simulink library "vmc"  (R2021b)
settings: Solver=VariableStepAuto  StartTime=0.0  StopTime=10.0  RelTol=1e-3
undefined symbols (not defined in the file or in its folder): AVMC_ACCDeltaTqIGain4OVRD_X_kph, AVMC_ACCDeltaTqIGain4OVRD_Y_mps2, AVMC_ACCDeltaTqIGain_X_kph, AVMC_ACCDeltaTqIGain_Y_mps2, AVMC_ACCDeltaTqPGain_X_kph, AVMC_ACCDeltaTqPGain_Y_kph, AVMC_ACCLongSteadyCtrl_X_kph, AVMC_ADSPosGFBDeltaTq_X_kph, AVMC_ADSPosGFBDeltaTq_Y_mps2, AVMC_AggressJerkPCT4AT_X_kph, AVMC_AggressJerkPCT_X_kph, AVMC_AggressLimitPCT4AT_X_kph, AVMC_AggressLimitPCT_X_kph, AVMC_CCLongSteadyCtrl_X_kph, AVMC_DISCDeltaTqIGain_X_kph, AVMC_DISCDeltaTqIGain_Y_mps2, AVMC_DISCDeltaTqPGain_X_kph, AVMC_DISCDeltaTqPGain_Y_kph, AVMC_ESCRegenOut_X_kph, AVMC_ESCRegenOut_Y_Deg, AVMC_ESCRegenOutEnSpd_X_Deg, AVMC_ISOAccLimit_X_mps, AVMC_ISODecLimit_X_mps, AVMC_ISOJerk_X_mps, AVMC_LatESCRegenOut_X_kph, AVMC_LatESCRegenOut_Y_Deg, AVMC_LongAccDeadZone_X_kph, AVMC_LongAccFiltTsforP2_X_Gps, AVMC_MCPresBaseTq_X_bar, AVMC_MSALongSteadyCtrl_X_kph, AVMC_MSAPedalOvrd_X_kph, AVMC_MSASpdBand_X_kph, AVMC_MSATqDownEndTq_X_kph, AVMC_MSATqDownTime_X_kph, AVMC_OPDDisSlideRate_X_Deg, AVMC_OVRD2ActSR2FCMCMD_X_mps2, AVMC_PedalTqRWhlRatio_X_Nm, AVMC_PedalTqRWhlRatio_Y_gps, AVMC_PedalTqRWhlSlipGain_X_rat, AVMC_PedalTqRWhlSlipGain_Y_kph, AVMC_PedalTqRWhSTRGGain_X_deg, AVMC_PedalTqRWhSTRGGain_Y_kph, AVMC_RDCDetectTime_X_kph, AVMC_RDCDetectTime_Y_pct, AVMC_RDCEnSlideRate_X_Deg, AVMC_RearWhlTqRatio_X_Nm, AVMC_RearWhlTqRatio_Y_gps, AVMC_RearWhlTqSlipGain_X_rat, AVMC_RearWhlTqSlipGain_Y_kph, AVMC_RearWhlTqSTRGGain_X_deg, AVMC_RearWhlTqSTRGGain_Y_kph, AVMC_ReqBrkJoinDecSR_X_mps2, AVMC_SoftJerkPCT_X_kph, AVMC_SoftLimitPCT_X_kph, AVMC_StESCYaw_X_kph, AVMC_StESCYaw_Y_Deg, AVMC_StESCYawCom_X_kph, AVMC_StESCYawCom_Y_Gps, AVMC_TMSpdBaseTq_X_rpm, AVMC_VehHoldDecCtrlTime2_X_kph ... (+411)
libraries: hcu_lib x108, simulink x82, tqr x1, simulink_extras x1
(part 12 of 14)

== system vmc/VMC/VMC/SpeedArbitration/Response Gain ==
  VDSC_DISCTurn_flg : Inport
  VVMC_FeatArbitrSta_enum : Inport  Port=2
  VVMC_FeatReqSpd_kph : Inport  Port=3
  VVMC_MeterIndSpeedForCalcu_kph : Inport  Port=4
  VINP_VehSpeed_kph : Inport  Port=5
  VDSC_AutoTurnMode_flg : Inport  Port=6
  VDSC_DISCTargetSpd_kph : Inport  Port=7
  Abs : Abs
  Add : Sum  Inputs=-+
  Add4 : Sum
  Constant1 : Constant  Value=KVMC_Veh2MeterSpdFactor_enum
  Constant13 : Constant  Value=ENUM_FEATARBITRSTA_DISC
  Constant{15,29,31,33,35} (5 alike) : Constant  Value=ZERO_FLOAT
  Constant16 : Constant  Value=ENUM_DISCTURN_ACTIVE
  Constant18 : Constant  Value=ENUM_FEATARBITRSTA_ACCDISC
  Constant2 : Constant  Value=ENUM_FEATARBITRSTA_CC
  Constant23 : Constant  Value=KVMC_Veh2MeterSpdOffset_enum
  Constant28 : Constant  Value=KVMC_Veh2MeterSpdLoFactor_enum
  Constant3 : Constant  Value=ENUM_FEATARBITRSTA_MSA
  Constant{30,32,34,36} (4 alike) : Constant  Value=HUNDRED
  Constant4 : Constant  Value=TRUE
  Constant5 : Constant  Value=KVMC_MSAResponseAGSV_flg
  Divide5 : Product  Inputs=**
  Divide8 : Product  Inputs=**
  MVMC_AggressJerkPCT4AT_pct : Lookup_n-D  NumberOfTableDimensions=1  BreakpointsForDimension1=AVMC_AggressJerkPCT4AT_X_kph  Table=MVMC_AggressJerkPCT4AT_Y_pct  InternalRulePriority=Speed  RndMeth=Simplest  InputSameDT=on
  MVMC_AggressJerkPCT_pct : Lookup_n-D  NumberOfTableDimensions=1  BreakpointsForDimension1=AVMC_AggressJerkPCT_X_kph  Table=MVMC_AggressJerkPCT_Y_pct  InternalRulePriority=Speed  RndMeth=Simplest  InputSameDT=on
  MVMC_AggressJerkPCT_pct1 : Lookup_n-D  NumberOfTableDimensions=1  BreakpointsForDimension1=AVMC_AggressJerkPCT_X_kph  Table=MVMC_AggressJerkPCT_Y_pct  InternalRulePriority=Speed  RndMeth=Simplest  InputSameDT=on
  MVMC_AggressLimitPCT4AT_pct : Lookup_n-D  NumberOfTableDimensions=1  BreakpointsForDimension1=AVMC_AggressLimitPCT4AT_X_kph  Table=MVMC_AggressLimitPCT4AT_Y_pct  InternalRulePriority=Speed  RndMeth=Simplest  InputSameDT=on
  MVMC_AggressLimitPCT_pct : Lookup_n-D  NumberOfTableDimensions=1  BreakpointsForDimension1=AVMC_AggressLimitPCT_X_kph  Table=MVMC_AggressLimitPCT_Y_pct  InternalRulePriority=Speed  RndMeth=Simplest  InputSameDT=on
  MVMC_AggressLimitPCT_pct1 : Lookup_n-D  NumberOfTableDimensions=1  BreakpointsForDimension1=AVMC_AggressLimitPCT_X_kph  Table=MVMC_AggressLimitPCT_Y_pct  InternalRulePriority=Speed  RndMeth=Simplest  InputSameDT=on
  MVMC_SoftJerkPCT_pct : Lookup_n-D  NumberOfTableDimensions=1  BreakpointsForDimension1=AVMC_SoftJerkPCT_X_kph  Table=MVMC_SoftJerkPCT_Y_pct  InternalRulePriority=Speed  RndMeth=Simplest  InputSameDT=on
  MVMC_SoftLimitPCT_pct : Lookup_n-D  NumberOfTableDimensions=1  BreakpointsForDimension1=AVMC_SoftLimitPCT_X_kph  Table=MVMC_SoftLimitPCT_Y_pct  InternalRulePriority=Speed  RndMeth=Simplest  InputSameDT=on
  Relational Operator : RelationalOperator  Operator=>  OutDataTypeStr=boolean  RndMeth=Simplest
  Relational Operator1 : RelationalOperator  Operator=>  OutDataTypeStr=boolean  RndMeth=Simplest
  Response Gain : Stateflow chart  TreatAsAtomicUnit=on
  Saturation Dynamic{1..4} (4 alike) : simulink/Discontinuities/Saturation Dynamic  OutMin=[]  OutMax=[]  OutDataTypeStr=Inherit: Same as second input  OutDataType=fixdt(1, 16)  OutScaling=2^-10  DoSatur=off
  Switch : Switch  Criteria=u2 > Threshold  Threshold=KVMC_Veh2MeterSpdLoBdy_kph
  Switch{1..4} (4 alike) : Switch  Criteria=u2 > Threshold
  VVMC_JerkPCT_pct : Outport
  VVMC_LimitPCT_pct : Outport  Port=2
  wires:
  Switch/1 -> Add/1
  VINP_VehSpeed_kph/1 -> [VINP_VehSpeed_kph]
  Abs/1 -> MVMC_SoftLimitPCT_pct/1, MVMC_AggressLimitPCT_pct/1, MVMC_AggressLimitPCT4AT_pct/1, MVMC_AggressLimitPCT_pct1/1
  Add/1 -> Abs/1
  [VVMC_FeatReqSpd_kph] -> Add/2
  VVMC_FeatReqSpd_kph/1 -> [VVMC_FeatReqSpd_kph]
  Switch1/1 -> Saturation Dynamic3/2
  Saturation Dynamic1/1 -> [VVMC_SoftLimitPCT_pct]  "VVMC_SoftLimitPCT_pct"
  Saturation Dynamic2/1 -> [VVMC_AggressJerkPCT_pct]  "VVMC_AggressJerkPCT_pct"
  Saturation Dynamic4/1 -> [VVMC_SoftJerkPCT_pct]  "VVMC_SoftJerkPCT_pct"
  [VVMC_MeterIndSpeedForCalcu_kph] -> MVMC_SoftJerkPCT_pct/1, MVMC_AggressJerkPCT4AT_pct/1, MVMC_AggressJerkPCT_pct/1, MVMC_AggressJerkPCT_pct1/1
  VVMC_MeterIndSpeedForCalcu_kph/1 -> [VVMC_MeterIndSpeedForCalcu_kph]
  Constant18/1 -> Response Gain/11(ENUM_FEATARBITRSTA_ACCDISC)
  Constant16/1 -> Response Gain/10(ENUM_DISCTURN_ACTIVE)
  Constant15/1 -> Response Gain/9(ZERO_FLOAT)
  Constant13/1 -> Response Gain/7(ENUM_FEATARBITRSTA_DISC)
  [VVMC_LimitPCT_pct] -> VVMC_LimitPCT_pct/1
  [VVMC_JerkPCT_pct] -> VVMC_JerkPCT_pct/1
  [VVMC_AggressLimitPCT_pct] -> Response Gain/6(VVMC_AggressLimitPCT_pct)
  [VVMC_SoftLimitPCT_pct] -> Response Gain/5(VVMC_SoftLimitPCT_pct)
  [VVMC_AggressJerkPCT_pct] -> Response Gain/4(VVMC_AggressJerkPCT_pct)
  [VVMC_SoftJerkPCT_pct] -> Response Gain/3(VVMC_SoftJerkPCT_pct)
  [VVMC_FeatArbitrSta_enum] -> Response Gain/2(VVMC_FeatArbitrSta_enum)
  VVMC_FeatArbitrSta_enum/1 -> [VVMC_FeatArbitrSta_enum]
  VDSC_DISCTurn_flg/1 -> [VDSC_DISCTurn_flg]
  Response Gain/2(VVMC_LimitPCT_pct) -> [VVMC_LimitPCT_pct]
  [VDSC_DISCTurn_flg] -> Response Gain/1(VDSC_DISCTurn_flg)
  Response Gain/1(VVMC_JerkPCT_pct) -> [VVMC_JerkPCT_pct]
  Constant23/1 -> Add4/1
  Divide8/1 -> Switch/3
  Constant28/1 -> Divide8/2
  Add4/1 -> Switch/1
  Divide5/1 -> Add4/2
  [VINP_VehSpeed_kph] -> Switch/2, Divide8/1, Divide5/2
  Constant1/1 -> Divide5/1
  Constant2/1 -> Response Gain/8(ENUM_FEATARBITRSTA_CC)
  Constant3/1 -> Response Gain/12(ENUM_FEATARBITRSTA_MSA)
  Constant4/1 -> Response Gain/13(TRUE)
  Constant5/1 -> Response Gain/14(KVMC_MSAResponseAGSV_flg)
  VDSC_AutoTurnMode_flg/1 -> [VDSC_AutoTurnMode_flg]
  [VDSC_AutoTurnMode_flg] -> Switch2/2
  MVMC_AggressJerkPCT4AT_pct/1 -> Switch4/3
  [VDSC_AutoTurnMode_flg] -> Switch1/2
  MVMC_AggressLimitPCT4AT_pct/1 -> Switch3/3
  VDSC_DISCTargetSpd_kph/1 -> [VDSC_DISCTargetSpd_kph]
  [VVMC_MeterIndSpeedForCalcu_kph] -> Relational Operator/2
  [VDSC_DISCTargetSpd_kph] -> Relational Operator/1
  Relational Operator/1 -> Switch3/2
  MVMC_AggressLimitPCT_pct1/1 -> Switch3/1
  Switch3/1 -> Switch1/1
  Switch4/1 -> Switch2/1
  MVMC_AggressJerkPCT_pct1/1 -> Switch4/1
  Relational Operator1/1 -> Switch4/2
  [VDSC_DISCTargetSpd_kph] -> Relational Operator1/1
  [VVMC_MeterIndSpeedForCalcu_kph] -> Relational Operator1/2
  MVMC_AggressLimitPCT_pct/1 -> Switch1/3
  MVMC_AggressJerkPCT_pct/1 -> Switch2/3
  Saturation Dynamic3/1 -> [VVMC_AggressLimitPCT_pct]  "VVMC_AggressLimitPCT_pct"
  Constant30/1 -> Saturation Dynamic3/1
  Constant29/1 -> Saturation Dynamic3/3
  Constant32/1 -> Saturation Dynamic1/1
  Constant31/1 -> Saturation Dynamic1/3
  MVMC_SoftLimitPCT_pct/1 -> Saturation Dynamic1/2
  Constant34/1 -> Saturation Dynamic2/1
  Constant33/1 -> Saturation Dynamic2/3
  Switch2/1 -> Saturation Dynamic2/2
  Constant36/1 -> Saturation Dynamic4/1
  Constant35/1 -> Saturation Dynamic4/3
  MVMC_SoftJerkPCT_pct/1 -> Saturation Dynamic4/2

== system vmc/VMC/VMC/ACC_Function/ACC Torque Source Determination/Triggered Subsystem2 ==
  In1 : Inport
  Trigger : TriggerPort  VariantControl=(inherit)
  Out1 : Outport
  wires:
  In1/1 -> Out1/1

== system vmc/VMC/VMC/ACC_Function/VVMC_ADASWhlTqCalVehHoldStandstill_Nm/Triggered Subsystem1 ==
  In1 : Inport
  In2 : Inport  Port=2
  Trigger : TriggerPort  VariantControl=(inherit)
  Out1 : Outport
  Out2 : Outport  Port=2
  wires:
  In1/1 -> Out1/1
  In2/1 -> Out2/1

== system vmc/VMC/VMC/ACC_Function/VVMC_ADASWhlTqCalVehHoldStandstill_Nm/Triggered Subsystem4 ==
  In1 : Inport
  Trigger : TriggerPort  VariantControl=(inherit)
  Out1 : Outport
  wires:
  In1/1 -> Out1/1

== system vmc/VMC/VMC/APS function/Signal Rounting1/Signal Determination VINP_APSDecReqAtest_flg ==
  SignalInput1 : Inport
  SignalInput2 : Inport  Port=2
  VINP_SCPSystemMode_enum : Inport  Port=3
  VVMC_APSActive_flg : Inport  Port=4
  VVMC_ADASActive_flg : Inport  Port=5
  VVMC_CAASActive_flg : Inport  Port=6
  AND : Logic  Inputs=3  AllPortsSameDT=off  OutDataTypeStr=boolean
  Constant1 : Constant  Value=ENUM_SYSMODE_PRODUCT
  Constant3 : Constant  Value=KVMC_APSDevelopeSW_flg
  Equal : RelationalOperator  Operator===  OutDataTypeStr=boolean  RndMeth=Simplest
  OR : Logic  Operator=OR  Inputs=3  AllPortsSameDT=off  OutDataTypeStr=boolean
  Switch : Switch  Criteria=u2 > Threshold
  SignalOutp : Outport
  wires:
  VVMC_ADASActive_flg/1 -> OR/2
  AND/1 -> OR/1
  OR/1 -> Switch/2
  VVMC_APSActive_flg/1 -> AND/3
  Equal/1 -> AND/1
  VINP_SCPSystemMode_enum/1 -> Equal/1
  Switch/1 -> SignalOutp/1
  SignalInput1/1 -> Switch/1
  SignalInput2/1 -> Switch/3
  Constant3/1 -> AND/2
  Constant1/1 -> Equal/2
  VVMC_CAASActive_flg/1 -> OR/3

== system vmc/VMC/VMC/APS function/Signal Rounting1/Signal Determination VINP_APSDecReqtest_mps2 ==
  SignalInput1 : Inport
  SignalInput2 : Inport  Port=2
  VINP_SCPSystemMode_enum : Inport  Port=3
  VVMC_APSActive_flg : Inport  Port=4
  VVMC_ADASActive_flg : Inport  Port=5
  VVMC_CAASActive_flg : Inport  Port=6
  AND : Logic  Inputs=3  AllPortsSameDT=off  OutDataTypeStr=boolean
  Constant1 : Constant  Value=ENUM_SYSMODE_PRODUCT
  Constant3 : Constant  Value=KVMC_APSDevelopeSW_flg
  Equal : RelationalOperator  Operator===  OutDataTypeStr=boolean  RndMeth=Simplest
  OR : Logic  Operator=OR  Inputs=3  AllPortsSameDT=off  OutDataTypeStr=boolean
  Switch : Switch  Criteria=u2 > Threshold
  SignalOutp : Outport
  wires:
  Constant1/1 -> Equal/2
  Constant3/1 -> AND/2
  SignalInput2/1 -> Switch/3
  SignalInput1/1 -> Switch/1
  Switch/1 -> SignalOutp/1
  VINP_SCPSystemMode_enum/1 -> Equal/1
  Equal/1 -> AND/1
  VVMC_APSActive_flg/1 -> AND/3
  OR/1 -> Switch/2
  AND/1 -> OR/1
  VVMC_ADASActive_flg/1 -> OR/2
  VVMC_CAASActive_flg/1 -> OR/3

== system vmc/VMC/VMC/APS function/Signal Rounting1/Signal Determination VINP_APSReqtest_enum ==
  SignalInput1 : Inport
  SignalInput2 : Inport  Port=2
  VINP_SCPSystemMode_enum : Inport  Port=3
  VVMC_APSActive_flg : Inport  Port=4
  VVMC_ADASActive_flg : Inport  Port=5
  VVMC_CAASActive_flg : Inport  Port=6
  AND : Logic  Inputs=3  AllPortsSameDT=off  OutDataTypeStr=boolean
  Constant1 : Constant  Value=ENUM_SYSMODE_PRODUCT
  Constant3 : Constant  Value=KVMC_APSDevelopeSW_flg
  Equal : RelationalOperator  Operator===  OutDataTypeStr=boolean  RndMeth=Simplest
  OR : Logic  Operator=OR  Inputs=3  AllPortsSameDT=off  OutDataTypeStr=boolean
  Switch : Switch  Criteria=u2 > Threshold
  SignalOutp : Outport
  wires:
  VVMC_ADASActive_flg/1 -> OR/2
  AND/1 -> OR/1
  OR/1 -> Switch/2
  VVMC_APSActive_flg/1 -> AND/3
  Equal/1 -> AND/1
  VINP_SCPSystemMode_enum/1 -> Equal/1
  Switch/1 -> SignalOutp/1
  SignalInput1/1 -> Switch/1
  SignalInput2/1 -> Switch/3
  Constant3/1 -> AND/2
  Constant1/1 -> Equal/2
  VVMC_CAASActive_flg/1 -> OR/3

== system vmc/VMC/VMC/APS function/Signal Rounting1/Signal Determination VINP_APSStaSystemtest_enum ==
  SignalInput1 : Inport
  SignalInput2 : Inport  Port=2
  VINP_SCPSystemMode_enum : Inport  Port=3
  VVMC_APSActive_flg : Inport  Port=4
  VVMC_ADASActive_flg : Inport  Port=5
  VTQD_GearActualPosn_enum : Inport  Port=6
  VVMC_CAASActive_flg : Inport  Port=7
  AND : Logic  Inputs=3  AllPortsSameDT=off  OutDataTypeStr=boolean
  AND1 : Logic  AllPortsSameDT=off  OutDataTypeStr=boolean
  Constant1 : Constant  Value=ENUM_SYSMODE_PRODUCT
  Constant2 : Constant  Value=ENUM_GEARACTUALPOSN_P
  Constant3 : Constant  Value=KVMC_APSDevelopeSW_flg
  Constant4 : Constant  Value=ENUM_APSSYSTEMSTA_ENABLE
  Constant5 : Constant  Value=KVMC_APSStaSystemOvrd_flg
  Equal : RelationalOperator  Operator===  OutDataTypeStr=boolean  RndMeth=Simplest
  Equal1 : RelationalOperator  Operator===  OutDataTypeStr=boolean  RndMeth=Simplest
  Equal2 : RelationalOperator  Operator===  OutDataTypeStr=boolean  RndMeth=Simplest
  OR : Logic  Operator=OR  Inputs=5  AllPortsSameDT=off  OutDataTypeStr=boolean
  Switch : Switch  Criteria=u2 > Threshold
  SignalOutp : Outport
  wires:
  Constant1/1 -> Equal/2
  Constant3/1 -> AND/2
  SignalInput2/1 -> Switch/3
  SignalInput1/1 -> Switch/1, [VINP_APSStaSystem_enum]
  Switch/1 -> SignalOutp/1
  VINP_SCPSystemMode_enum/1 -> Equal/1
  Equal/1 -> AND/1
  VVMC_APSActive_flg/1 -> AND/3
  OR/1 -> Switch/2
  AND/1 -> OR/1
  VVMC_ADASActive_flg/1 -> OR/2
  VTQD_GearActualPosn_enum/1 -> Equal1/1
  Constant2/1 -> Equal1/2
  Equal1/1 -> AND1/1
  Equal2/1 -> AND1/2
  [VINP_APSStaSystem_enum] -> Equal2/1
  Constant4/1 -> Equal2/2
  AND1/1 -> OR/3
  Constant5/1 -> OR/4
  VVMC_CAASActive_flg/1 -> OR/5

== system vmc/VMC/VMC/MSA function/MSADemandTorqueCalculation/Triggered Subsystem ==
  In1 : Inport
  Trigger : TriggerPort  VariantControl=(inherit)
  Out1 : Outport
  wires:
  In1/1 -> Out1/1

== system vmc/VMC/VMC/MSA function/MSATorqueSourceDetermination/Triggered Subsystem2 ==
  In1 : Inport
  Trigger : TriggerPort  VariantControl=(inherit)
  Out1 : Outport
  wires:
  In1/1 -> Out1/1

== system vmc/VMC/VMC/SPD2ACC/VVMC_DISReqAcc_mps2/Triggered Subsystem4 ==
  In1 : Inport
  Trigger : TriggerPort  VariantControl=(inherit)
  Out1 : Outport
  wires:
  In1/1 -> Out1/1

== system vmc/VMC/VMC/SPD2ACC/VVMC_DISReqAcc_mps2/Triggered Subsystem6 ==
  In1 : Inport
  In2 : Inport  Port=2
  In3 : Inport  Port=3
  Trigger : TriggerPort  VariantControl=(inherit)
  Out1 : Outport
  Out2 : Outport  Port=2
  Out3 : Outport  Port=3
  wires:
  In1/1 -> Out1/1
  In2/1 -> Out2/1
  In3/1 -> Out3/1

== system vmc/VMC/VMC/SPD2ACC/VVMC_DISReqAcc_mps2/Triggered Subsystem7 ==
  In1 : Inport
  Trigger : TriggerPort  VariantControl=(inherit)
  Out1 : Outport
  wires:
  In1/1 -> Out1/1

== system vmc/VMC/VMC/SafetyControl/SafetyControlJudgement/FrontRearSlipRatio ==
  VVMC_LFWhlSpeedRollAve_kph : Inport
  VVMC_RFWhlSpeedRollAve_kph : Inport  Port=2
  VVMC_LRWhlSpeedRollAve_kph : Inport  Port=3
  VVMC_RRWhlSpeedRollAve_kph : Inport  Port=4
  VINP_LFRawWhlSpeedV_flg : Inport  Port=5
  VINP_RFRawWhlSpeedV_flg : Inport  Port=6
  VINP_LRRawWhlSpeedV_flg : Inport  Port=7
  VINP_RRRawWhlSpeedV_flg : Inport  Port=8
  Constant : Constant  Value=KVMC_FrontRearSlipRatioTHR_kph
  Constant1 : Constant  Value=TRUE
  Constant2 : Constant  Value=FALSE
  Constant3 : Constant  Value=TWO_FLOAT
  Constant4 : Constant  Value=ZERO_FLOAT
  FrontRearSlipRatioJudgement : Stateflow chart  TreatAsAtomicUnit=on
  "VVMC_FrontRearSlipRatioCtrl_flg " : Outport
  wires:
  Constant4/1 -> FrontRearSlipRatioJudgement/13(ZERO_FLOAT)
  Constant3/1 -> FrontRearSlipRatioJudgement/12(TWO_FLOAT)
  Constant2/1 -> FrontRearSlipRatioJudgement/11(FALSE)
  [VVMC_FrontRearSlipRatioCtrl_flg] -> "VVMC_FrontRearSlipRatioCtrl_flg "/1
  FrontRearSlipRatioJudgement/1(VVMC_FrontRearSlipRatioCtrl_flg) -> [VVMC_FrontRearSlipRatioCtrl_flg]
  Constant1/1 -> FrontRearSlipRatioJudgement/10(TRUE)
  Constant/1 -> FrontRearSlipRatioJudgement/9(KVMC_FrontRearSlipRatioTHR_kph)
  [VINP_RRRawWhlSpeedV_flg] -> FrontRearSlipRatioJudgement/8(VINP_RRRawWhlSpeedV_flg)
  [VVMC_RRWhlSpeedRollAve_kph] -> FrontRearSlipRatioJudgement/4(VVMC_RRWhlSpeedRollAve_kph)
  [VVMC_RFWhlSpeedRollAve_kph] -> FrontRearSlipRatioJudgement/2(VVMC_RFWhlSpeedRollAve_kph)
  [VVMC_LFWhlSpeedRollAve_kph] -> FrontRearSlipRatioJudgement/1(VVMC_LFWhlSpeedRollAve_kph)
  [VINP_RFRawWhlSpeedV_flg] -> FrontRearSlipRatioJudgement/6(VINP_RFRawWhlSpeedV_flg)
  [VVMC_LRWhlSpeedRollAve_kph] -> FrontRearSlipRatioJudgement/3(VVMC_LRWhlSpeedRollAve_kph)
  [VINP_LFRawWhlSpeedV_flg] -> FrontRearSlipRatioJudgement/5(VINP_LFRawWhlSpeedV_flg)
  [VINP_LRRawWhlSpeedV_flg] -> FrontRearSlipRatioJudgement/7(VINP_LRRawWhlSpeedV_flg)
  VINP_RRRawWhlSpeedV_flg/1 -> [VINP_RRRawWhlSpeedV_flg]
  VINP_LRRawWhlSpeedV_flg/1 -> [VINP_LRRawWhlSpeedV_flg]
  VINP_RFRawWhlSpeedV_flg/1 -> [VINP_RFRawWhlSpeedV_flg]
  VINP_LFRawWhlSpeedV_flg/1 -> [VINP_LFRawWhlSpeedV_flg]
  VVMC_RRWhlSpeedRollAve_kph/1 -> [VVMC_RRWhlSpeedRollAve_kph]
  VVMC_LRWhlSpeedRollAve_kph/1 -> [VVMC_LRWhlSpeedRollAve_kph]
  VVMC_RFWhlSpeedRollAve_kph/1 -> [VVMC_RFWhlSpeedRollAve_kph]
  VVMC_LFWhlSpeedRollAve_kph/1 -> [VVMC_LFWhlSpeedRollAve_kph]

== system vmc/VMC/VMC/SafetyControl/SafetyControlJudgement/LateralAccelerationControl ==
  VVMC_LatAccRollAve_Gps : Inport
  VINP_LatAccelV_flg : Inport  Port=2
  Abs : Abs
  Constant : Constant  Value=KVMC_LatAccCtrlTHR_Gps
  Logical Operator : Logic  Operator=OR  AllPortsSameDT=off  OutDataTypeStr=boolean
  Relational Operator : RelationalOperator  OutDataTypeStr=boolean  RndMeth=Simplest
  VVMC_LatAccCtrl_flg : Outport
  wires:
  Abs/1 -> Relational Operator/1
  Logical Operator/1 -> [VVMC_LatAccCtrl_flg]  "VVMC_LatAccCtrl_flg"
  [VINP_LatAccelV_flg] -> Logical Operator/2
  Relational Operator/1 -> Logical Operator/1
  Constant/1 -> Relational Operator/2
  [VVMC_LatAccRollAve_Gps] -> Abs/1
  [VVMC_LatAccCtrl_flg] -> VVMC_LatAccCtrl_flg/1
  VINP_LatAccelV_flg/1 -> [VINP_LatAccelV_flg]
  VVMC_LatAccRollAve_Gps/1 -> [VVMC_LatAccRollAve_Gps]

== system vmc/VMC/VMC/SafetyControl/SafetyControlJudgement/RearWheelSlipRatio ==
  VVMC_LRWhlSpeedRollAve_kph : Inport
  VVMC_RRWhlSpeedRollAve_kph : Inport  Port=2
  VINP_LRRawWhlSpeedV_flg : Inport  Port=3
  VINP_RRRawWhlSpeedV_flg : Inport  Port=4
  Constant : Constant  Value=KVMC_RearWhlSlipRatioTHR_kph
  Constant1 : Constant  Value=TRUE
  Constant2 : Constant  Value=FALSE
  FrontRearSlipRatioJudgement : Stateflow chart  TreatAsAtomicUnit=on
  "VVMC_RearWhlSlipRatioCtrl_flg " : Outport
  wires:
  VVMC_LRWhlSpeedRollAve_kph/1 -> [VVMC_LRWhlSpeedRollAve_kph]
  VVMC_RRWhlSpeedRollAve_kph/1 -> [VVMC_RRWhlSpeedRollAve_kph]
  VINP_LRRawWhlSpeedV_flg/1 -> [VINP_LRRawWhlSpeedV_flg]
  VINP_RRRawWhlSpeedV_flg/1 -> [VINP_RRRawWhlSpeedV_flg]
  [VINP_LRRawWhlSpeedV_flg] -> FrontRearSlipRatioJudgement/3(VINP_LRRawWhlSpeedV_flg)
  [VVMC_LRWhlSpeedRollAve_kph] -> FrontRearSlipRatioJudgement/1(VVMC_LRWhlSpeedRollAve_kph)
  [VVMC_RRWhlSpeedRollAve_kph] -> FrontRearSlipRatioJudgement/2(VVMC_RRWhlSpeedRollAve_kph)
  [VINP_RRRawWhlSpeedV_flg] -> FrontRearSlipRatioJudgement/4(VINP_RRRawWhlSpeedV_flg)
  Constant/1 -> FrontRearSlipRatioJudgement/5(KVMC_RearWhlSlipRatioTHR_kph)
  Constant1/1 -> FrontRearSlipRatioJudgement/6(TRUE)
  FrontRearSlipRatioJudgement/1(VVMC_RearWhlSlipRatioCtrl_flg) -> [VVMC_RearWhlSlipRatioCtrl_flg]
  [VVMC_RearWhlSlipRatioCtrl_flg] -> "VVMC_RearWhlSlipRatioCtrl_flg "/1
  Constant2/1 -> FrontRearSlipRatioJudgement/7(FALSE)

== system vmc/VMC/VMC/SafetyControl/SafetyControlJudgement/SafetyControlJudgement ==
  VVMC_FrontRearSlipRatioCtrl_flg : Inport
  VVMC_RearWhlSlipRatioCtrl_flg : Inport  Port=2
  VVMC_SingleWhlSlipRatioCtrl_flg : Inport  Port=3
  VVMC_LatAccCtrl_flg : Inport  Port=4
  VVMC_FeatArbitrFinal_enum : Inport  Port=5
  AND : Logic  AllPortsSameDT=off  OutDataTypeStr=boolean
  Constant1 : Constant  Value=KVMC_SafetyCtrlForACCSW_flg
  Constant17 : Constant  Value=ENUM_FEATARBITRSTA_DISC
  Constant2 : Constant  Value=ENUM_FEATARBITRSTA_ACC
  Logical Operator : Logic  Operator=OR  Inputs=4  AllPortsSameDT=off  OutDataTypeStr=boolean
  Logical Operator1 : Logic  AllPortsSameDT=off  OutDataTypeStr=boolean
  OR : Logic  Operator=OR  AllPortsSameDT=off  OutDataTypeStr=boolean
  Relational Operator : RelationalOperator  Operator===  OutDataTypeStr=boolean  RndMeth=Simplest
  Relational Operator1 : RelationalOperator  Operator===  OutDataTypeStr=boolean  RndMeth=Simplest
  "VVMC_SafetyCtrl_flg " : Outport
  wires:
  [VVMC_FeatArbitrFinal_enum] -> Relational Operator/1
  Relational Operator/1 -> OR/1
  Logical Operator/1 -> Logical Operator1/1
  Constant17/1 -> Relational Operator/2
  VVMC_FeatArbitrFinal_enum/1 -> [VVMC_FeatArbitrFinal_enum]
  [VVMC_LatAccCtrl_flg] -> Logical Operator/4
  VVMC_LatAccCtrl_flg/1 -> [VVMC_LatAccCtrl_flg]
  Logical Operator1/1 -> [VVMC_SafetyCtrl_flg]
  [VVMC_SingleWhlSlipRatioCtrl_flg] -> Logical Operator/3
  [VVMC_RearWhlSlipRatioCtrl_flg] -> Logical Operator/2
  [VVMC_FrontRearSlipRatioCtrl_flg] -> Logical Operator/1
  [VVMC_SafetyCtrl_flg] -> "VVMC_SafetyCtrl_flg "/1
  VVMC_SingleWhlSlipRatioCtrl_flg/1 -> [VVMC_SingleWhlSlipRatioCtrl_flg]
  VVMC_RearWhlSlipRatioCtrl_flg/1 -> [VVMC_RearWhlSlipRatioCtrl_flg]
  VVMC_FrontRearSlipRatioCtrl_flg/1 -> [VVMC_FrontRearSlipRatioCtrl_flg]
  Constant2/1 -> Relational Operator1/2
  [VVMC_FeatArbitrFinal_enum] -> Relational Operator1/1
  Relational Operator1/1 -> AND/1
  Constant1/1 -> AND/2
  AND/1 -> OR/2
  OR/1 -> Logical Operator1/2

== system vmc/VMC/VMC/SafetyControl/SafetyControlJudgement/SingleWheelSlipRatio ==
  VINP_VehSpeed_kph : Inport
  VVMC_LFWhlSpeedRollAve_kph : Inport  Port=2
  VVMC_RFWhlSpeedRollAve_kph : Inport  Port=3
  VVMC_LRWhlSpeedRollAve_kph : Inport  Port=4
  VVMC_RRWhlSpeedRollAve_kph : Inport  Port=5
  VINP_LFRawWhlSpeedV_flg : Inport  Port=6
  VINP_RFRawWhlSpeedV_flg : Inport  Port=7
  VINP_LRRawWhlSpeedV_flg : Inport  Port=8
  VINP_RRRawWhlSpeedV_flg : Inport  Port=9
  Constant : Constant  Value=KVMC_SingleWhlSlipRatioTHR_kph
  Constant1 : Constant  Value=TRUE
  Constant2 : Constant  Value=FALSE
  SingleWheelSlipRatioJudgement : Stateflow chart  TreatAsAtomicUnit=on
  VVMC_SingleWhlSlipRatioCtrl_flg : Outport
  wires:
  [VINP_VehSpeed_kph] -> SingleWheelSlipRatioJudgement/1(VINP_VehSpeed_kph)
  VINP_VehSpeed_kph/1 -> [VINP_VehSpeed_kph]
  VVMC_LFWhlSpeedRollAve_kph/1 -> [VVMC_LFWhlSpeedRollAve_kph]
  VVMC_RFWhlSpeedRollAve_kph/1 -> [VVMC_RFWhlSpeedRollAve_kph]
  VVMC_LRWhlSpeedRollAve_kph/1 -> [VVMC_LRWhlSpeedRollAve_kph]
  VVMC_RRWhlSpeedRollAve_kph/1 -> [VVMC_RRWhlSpeedRollAve_kph]
  VINP_LFRawWhlSpeedV_flg/1 -> [VINP_LFRawWhlSpeedV_flg]
  VINP_RFRawWhlSpeedV_flg/1 -> [VINP_RFRawWhlSpeedV_flg]
  VINP_LRRawWhlSpeedV_flg/1 -> [VINP_LRRawWhlSpeedV_flg]
  VINP_RRRawWhlSpeedV_flg/1 -> [VINP_RRRawWhlSpeedV_flg]
  [VINP_LRRawWhlSpeedV_flg] -> SingleWheelSlipRatioJudgement/8(VINP_LRRawWhlSpeedV_flg)
  [VINP_LFRawWhlSpeedV_flg] -> SingleWheelSlipRatioJudgement/6(VINP_LFRawWhlSpeedV_flg)
  [VVMC_LRWhlSpeedRollAve_kph] -> SingleWheelSlipRatioJudgement/4(VVMC_LRWhlSpeedRollAve_kph)
  [VINP_RFRawWhlSpeedV_flg] -> SingleWheelSlipRatioJudgement/7(VINP_RFRawWhlSpeedV_flg)
  [VVMC_LFWhlSpeedRollAve_kph] -> SingleWheelSlipRatioJudgement/2(VVMC_LFWhlSpeedRollAve_kph)
  [VVMC_RFWhlSpeedRollAve_kph] -> SingleWheelSlipRatioJudgement/3(VVMC_RFWhlSpeedRollAve_kph)
  [VVMC_RRWhlSpeedRollAve_kph] -> SingleWheelSlipRatioJudgement/5(VVMC_RRWhlSpeedRollAve_kph)
  [VINP_RRRawWhlSpeedV_flg] -> SingleWheelSlipRatioJudgement/9(VINP_RRRawWhlSpeedV_flg)
  Constant/1 -> SingleWheelSlipRatioJudgement/10(KVMC_SingleWhlSlipRatioTHR_kph)
  Constant1/1 -> SingleWheelSlipRatioJudgement/11(TRUE)
  SingleWheelSlipRatioJudgement/1(VVMC_SingleWhlSlipRatioCtrl_flg) -> [VVMC_SingleWhlSlipRatioCtrl_flg]
  [VVMC_SingleWhlSlipRatioCtrl_flg] -> VVMC_SingleWhlSlipRatioCtrl_flg/1
  Constant2/1 -> SingleWheelSlipRatioJudgement/12(FALSE)

== system vmc/VMC/VMC/Slide Rate  Calculation/4Wheel Calculation/Determination ==
  VVMC_4WheelLongAcc_Gps : Inport
  task_time_s : Inport  Port=2
  VINP_VehSpeed_kph : Inport  Port=3
  VTQD_GearActualPosn_enum : Inport  Port=4
  VVMC_LFWhlSkid_flg : Inport  Port=5
  VVMC_RFWhlSkid_flg : Inport  Port=6
  VVMC_LRWhlSkid_flg : Inport  Port=7
  VVMC_RRWhlSkid_flg : Inport  Port=8
  VVMC_LF4WhlSpdSlideRate_pct : Inport  Port=9
  VVMC_RF4WhlSpdSlideRate_pct : Inport  Port=10
  VVMC_LR4WhlSpdSlideRate_pct : Inport  Port=11
  VVMC_RR4WhlSpdSlideRate_pct : Inport  Port=12
  VTQD_AfterAvailableTqDemFr_Nm : Inport  Port=13
  VTQD_AfterAvailableTqDemRr_Nm : Inport  Port=14
  VVMC_LFPreVehSpd_kph : Inport  Port=15
  VVMC_RFPreVehSpd_kph : Inport  Port=16
  VVMC_LRPreVehSpd_kph : Inport  Port=17
  VVMC_RRPreVehSpd_kph : Inport  Port=18
  AND : Logic  Inputs=4  AllPortsSameDT=off  OutDataTypeStr=boolean
  Add : Sum
  Add1 : Sum  Inputs=++++
  Add17 : Sum
  Add2 : Sum
  Constant1 : Constant  Value=GRAVITY_G
  Constant10 : Constant  Value=3
  Constant11 : Constant  Value=KPH2MPS
  Constant2 : Constant  Value=MPS2KPH
  Constant3 : Constant  Value=KVMC_PreVehSpdNum_c
  Constant4 : Constant  Value=ZERO_FLOAT
  Constant44 : Constant  Value=KPH2MPS
  Constant45 : Constant  Value=ZERO_FLOAT
  Constant46 : Constant  Value=ENUM_GEARACTUALPOSN_D
  Constant47 : Constant  Value=ENUM_GEARACTUALPOSN_R
  Constant48 : Constant  Value=KVMC_PreVehSpdCalSW_flg
  Constant5 : Constant  Value=KVMC_PreVehSpdSource_enum
  Constant6 : Constant
  Constant7 : Constant  Value=KVMC_PreVehSpdSource_enum
  Constant8 : Constant  Value=2
  Constant9 : Constant  Value=KVMC_PreVehSpdSource_enum
  Delay : Delay  DelayLength=1
  Delay5 : Delay  DelayLength=1
  Divide : Product  Inputs=*/
  Equal{,1..4} (5 alike) : RelationalOperator  Operator===  OutDataTypeStr=boolean  RndMeth=Simplest
  Max : MinMax  Function=max  Inputs=4
  Max1 : MinMax  Inputs=4
  Max2 : MinMax  Function=max  Inputs=4
  Max3 : MinMax  Inputs=4
  OR : Logic  Operator=OR  AllPortsSameDT=off  OutDataTypeStr=boolean
  OR1 : Logic  Operator=OR  AllPortsSameDT=off  OutDataTypeStr=boolean
  Product : Product
  Product1 : Product  Inputs=3
  Product2 : Product
  Product3 : Product
  Relational Operator1 : RelationalOperator  Operator=<=  OutDataTypeStr=boolean  RndMeth=Simplest
  Relational Operator16 : RelationalOperator  Operator=<=  OutDataTypeStr=boolean  RndMeth=Simplest
  Saturation : Saturate  UpperLimit=KVMC_PredVehSpdLimit_mps  LowerLimit=ZERO_FLOAT
  Switch{,1..4,9..10} (7 alike) : Switch  Criteria=u2 > Threshold
  VVMC_PredictVehSpd_kph : Outport
  VVMC_AllWhlSkid_flg : Outport  Port=2
  VVMC_4WhlSpdSlideRate_pct : Outport  Port=3
  wires:
  [VVMC_RRWhlSkid_flg] -> AND/4
  Add/1 -> Product2/1  "VVMC_CalPredictVehSpd_mps"
  Product2/1 -> Switch10/1
  Relational Operator16/1 -> Switch9/2
  [VVMC_LRWhlSkid_flg] -> AND/3
  Constant45/1 -> Relational Operator16/2
  Switch9/1 -> [VVMC_4WhlSpdSlideRate_pct]  "VVMC_4WhlSpdSlideRate_pct"
  Constant11/1 -> Product/2
  [VVMC_LFWhlSkid_flg] -> AND/1
  [VTQD_GearActualPosn_enum] -> Equal1/1
  Constant2/1 -> Product2/2
  Equal/1 -> OR/1
  AND/1 -> [VVMC_AllWhlSkid_flg]  "VVMC_AllWhlSkid_flg"
  Switch10/1 -> [VVMC_PredictVehSpd1_kph]  "VVMC_PredictVehSpd1_kph"
  Constant1/1 -> Product1/2
  [VINP_VehSpeed_kph] -> Switch10/3
  [VVMC_RF4WhlSpdSlideRate_pct] -> Max/2
  [VINP_VehSpeed_kph] -> Delay/1
  [task_time_s] -> Product1/3
  [VVMC_AllWhlSkid_flg] -> OR1/1
  [VVMC_RR4WhlSpdSlideRate_pct] -> Max/4
  OR/1 -> Switch10/2
  Switch/1 -> Saturation/1  "VVMC_LastPredictVehSpd_mps"
  Product/1 -> Switch/3
  Product3/1 -> Switch/1
  Delay5/1 -> Product3/1
  [VVMC_LR4WhlSpdSlideRate_pct] -> Max/3
  [VVMC_4WheelLongAcc_Gps] -> Product1/1
  [VVMC_LF4WhlSpdSlideRate_pct] -> Max1/1
  [VTQD_AfterAvailableTqDemRr_Nm] -> Add17/2
  [VVMC_LF4WhlSpdSlideRate_pct] -> Max/1
  [VVMC_RFWhlSkid_flg] -> AND/2
  [VVMC_Max4WhlSpdSlideRate_pct] -> Switch9/3
  Max1/1 -> [VVMC_Min4WhlSpdSlideRate_pct]  "VVMC_Min4WhlSpdSlideRate_pct"
  Saturation/1 -> Add/2
  [VTQD_GearActualPosn_enum] -> Equal/1
  [VVMC_RR4WhlSpdSlideRate_pct] -> Max1/4
  [VTQD_AfterAvailableTqDemFr_Nm] -> Add17/1
  OR1/1 -> Switch/2
  Product1/1 -> Add/1  "VVMC_DeltaVehSpd_mps"
  Constant46/1 -> Equal/2
  Delay/1 -> Product/1
  [VVMC_RF4WhlSpdSlideRate_pct] -> Max1/2
  Equal1/1 -> OR/2
  [VVMC_Min4WhlSpdSlideRate_pct] -> Switch9/1
  Constant47/1 -> Equal1/2
  Add17/1 -> Relational Operator16/1
  Max/1 -> [VVMC_Max4WhlSpdSlideRate_pct]  "VVMC_Max4WhlSpdSlideRate_pct"
  Constant44/1 -> Product3/2
  Constant48/1 -> OR1/2
  [VVMC_LR4WhlSpdSlideRate_pct] -> Max1/3
  VINP_VehSpeed_kph/1 -> [VINP_VehSpeed_kph]
  task_time_s/1 -> [task_time_s]
  VVMC_4WheelLongAcc_Gps/1 -> [VVMC_4WheelLongAcc_Gps]
  VTQD_GearActualPosn_enum/1 -> [VTQD_GearActualPosn_enum]
  [VVMC_PredictVehSpd_kph] -> VVMC_PredictVehSpd_kph/1
  [VVMC_AllWhlSkid_flg] -> VVMC_AllWhlSkid_flg/1
  [VVMC_4WhlSpdSlideRate_pct] -> VVMC_4WhlSpdSlideRate_pct/1
  VVMC_LFWhlSkid_flg/1 -> [VVMC_LFWhlSkid_flg]
  VVMC_RFWhlSkid_flg/1 -> [VVMC_RFWhlSkid_flg]
  VVMC_LRWhlSkid_flg/1 -> [VVMC_LRWhlSkid_flg]
  VVMC_RRWhlSkid_flg/1 -> [VVMC_RRWhlSkid_flg]
  VVMC_LF4WhlSpdSlideRate_pct/1 -> [VVMC_LF4WhlSpdSlideRate_pct]
  VVMC_RF4WhlSpdSlideRate_pct/1 -> [VVMC_RF4WhlSpdSlideRate_pct]
  VVMC_LR4WhlSpdSlideRate_pct/1 -> [VVMC_LR4WhlSpdSlideRate_pct]
  VVMC_RR4WhlSpdSlideRate_pct/1 -> [VVMC_RR4WhlSpdSlideRate_pct]
  VTQD_AfterAvailableTqDemFr_Nm/1 -> [VTQD_AfterAvailableTqDemFr_Nm]
  VTQD_AfterAvailableTqDemRr_Nm/1 -> [VTQD_AfterAvailableTqDemRr_Nm]
  VVMC_LFPreVehSpd_kph/1 -> [VVMC_LFPreVehSpd_kph]
  VVMC_RFPreVehSpd_kph/1 -> [VVMC_RFPreVehSpd_kph]
  VVMC_LRPreVehSpd_kph/1 -> [VVMC_LRPreVehSpd_kph]
  VVMC_RRPreVehSpd_kph/1 -> [VVMC_RRPreVehSpd_kph]
  [VVMC_LFPreVehSpd_kph] -> Add1/1
  [VVMC_RFPreVehSpd_kph] -> Add1/2
  [VVMC_LRPreVehSpd_kph] -> Add1/3
  [VVMC_RRPreVehSpd_kph] -> Add1/4
  Add1/1 -> Divide/1
  Constant3/1 -> Divide/2
  Divide/1 -> [VVMC_PredictVehSpd2_kph]  "VVMC_PredictVehSpd2_kph"
  [VVMC_LFPreVehSpd_kph] -> Max2/1
  [VVMC_RFPreVehSpd_kph] -> Max2/2
  [VVMC_LRPreVehSpd_kph] -> Max2/3
  [VVMC_RRPreVehSpd_kph] -> Max2/4
  Max2/1 -> [VVMC_Max4WhlPreVehSpd_kph]  "VVMC_Max4WhlPreVehSpd_kph"
  [VVMC_RRPreVehSpd_kph] -> Max3/4
  [VVMC_LRPreVehSpd_kph] -> Max3/3
  [VVMC_RFPreVehSpd_kph] -> Max3/2
  [VVMC_LFPreVehSpd_kph] -> Max3/1
  Max3/1 -> [VVMC_Min4WhlPreVehSpd_kph]  "VVMC_Min4WhlPreVehSpd_kph"
  Relational Operator1/1 -> Switch1/2
  Constant4/1 -> Relational Operator1/2
  Add2/1 -> Relational Operator1/1
  Switch1/1 -> [VVMC_PredictVehSpd3_kph]  "VVMC_PredictVehSpd3_kph"
  [VVMC_PredictVehSpd1_kph] -> Delay5/1
  Constant5/1 -> Equal2/1
  Constant6/1 -> Equal2/2
  Equal2/1 -> Switch2/2
  [VVMC_PredictVehSpd1_kph] -> Switch2/1
  [VINP_VehSpeed_kph] -> Switch2/3
  Equal3/1 -> Switch3/2
  Constant8/1 -> Equal3/2
  Constant7/1 -> Equal3/1
  Switch2/1 -> Switch3/3
  [VVMC_PredictVehSpd2_kph] -> Switch3/1
  Switch3/1 -> Switch4/3
  Constant9/1 -> Equal4/1
  Constant10/1 -> Equal4/2
  Equal4/1 -> Switch4/2
  [VVMC_PredictVehSpd3_kph] -> Switch4/1
  Switch4/1 -> [VVMC_PredictVehSpd_kph]  "VVMC_PredictVehSpd_kph"
  [VTQD_AfterAvailableTqDemFr_Nm] -> Add2/1
  [VTQD_AfterAvailableTqDemRr_Nm] -> Add2/2
  [VVMC_Max4WhlPreVehSpd_kph] -> Switch1/1
  [VVMC_Min4WhlPreVehSpd_kph] -> Switch1/3

== system vmc/VMC/VMC/Slide Rate  Calculation/4Wheel Calculation/LF Wheel ==
  VVMC_4WheelLongAcc_Gps : Inport
  task_time_s : Inport  Port=2
  VINP_LFRawWhlSpeed_kph : Inport  Port=3
  VTQD_GearActualPosn_enum : Inport  Port=4
  AND1 : Logic  Inputs=3  AllPortsSameDT=off  OutDataTypeStr=boolean
  Abs : Abs
  Add : Sum
  Add{1,5,9..10} (4 alike) : Sum  Inputs=+-
  Constant1 : Constant  Value=GRAVITY_G
  Constant11 : Constant  Value=KPH2MPS
  Constant2 : Constant  Value=MPS2KPH
  Constant24 : Constant  Value=KPH2MPS
  Constant25 : Constant  Value=GRAVITY_G
  Constant26 : Constant  Value=KVMC_WhlSpdCalAccTs_c
  Constant3 : Constant  Value=KVMC_4WheelEnSkidDetSpd_kph
  Constant36 : Constant  Value=KVMC_WheelSkidAccDev_Gps
  Constant37 : Constant  Value=KVMC_SkidRecVehSpdDev_kph
  Constant44 : Constant  Value=KPH2MPS
  Constant46 : Constant  Value=ENUM_GEARACTUALPOSN_D
  Constant47 : Constant  Value=ENUM_GEARACTUALPOSN_R
  Constant48 : Constant  Value=KVMC_PreVehSpdCalSW_flg
  Constant5 : Constant  Value=KVMC_RawWhlSpeedDeadZone_kph
  Constant52 : Constant  Value=KVMC_LFWhlSkidReset_flg
  Constant6 : Constant  Value=ONE_FLOAT
  Constant7 : Constant  Value=ONE_PERCENT
  Constant8 : Constant  Value=KVMC_RawWhlSpeedDeadZone_kph
  Constant9 : Constant  Value=ZERO_FLOAT
  Delay{,1,5..7,14} (6 alike) : Delay  DelayLength=1
  Divide : Product  Inputs=**//
  Divide1 : Product  Inputs=*//
  Equal : RelationalOperator  Operator===  OutDataTypeStr=boolean  RndMeth=Simplest
  Equal1 : RelationalOperator  Operator===  OutDataTypeStr=boolean  RndMeth=Simplest
  FirstOrderFilter : hcu_lib/Basic_Blocks/FirstOrderFilter
  OR : Logic  Operator=OR  AllPortsSameDT=off  OutDataTypeStr=boolean
  OR1 : Logic  Operator=OR  AllPortsSameDT=off  OutDataTypeStr=boolean
  OR2 : Logic  Operator=OR  AllPortsSameDT=off  OutDataTypeStr=boolean
  Product : Product
  Product1 : Product  Inputs=3
  Product2 : Product
  Product3 : Product
  Relational Operator : RelationalOperator  Operator=>  OutDataTypeStr=boolean  RndMeth=Simplest
  Relational Operator{1..3,9} (4 alike) : RelationalOperator  Operator=<=  OutDataTypeStr=boolean  RndMeth=Simplest
  SR_Latch : hcu_lib/Basic_Blocks/SR_Latch
  Saturation : Saturate  UpperLimit=KVMC_PredVehSpdLimit_mps  LowerLimit=ZERO_FLOAT
  Switch{,2..3,10} (4 alike) : Switch  Criteria=u2 > Threshold
  VVMC_LFPreVehSpd_kph : Outport
  VVMC_LFWhlSkid_flg : Outport  Port=2
  VVMC_LF4WhlSpdSlideRate_pct : Outport  Port=3
  wires:
  [VINP_LFRawWhlSpeed_kph] -> Delay7/1
  Constant37/1 -> Relational Operator9/2
  Relational Operator9/1 -> AND1/1
  Constant9/1 -> Switch3/1
  Constant36/1 -> Relational Operator/2
  Constant52/1 -> AND1/3
  Constant8/1 -> Relational Operator3/2
  Constant6/1 -> Switch2/1
  Delay14/1 -> AND1/2
  Abs/1 -> Relational Operator9/1
  [VVMC_4WheelLongAcc_Gps] -> Add9/2
  [VVMC_LFWhlSkid_flg] -> Delay14/1
  Relational Operator3/1 -> Switch3/2
  Add10/1 -> Abs/1
  [task_time_s] -> FirstOrderFilter/2
  Constant26/1 -> FirstOrderFilter/3
  Delay6/1 -> Add10/1
  SR_Latch/1 -> [VVMC_LFWhlSkid_flg]  "VVMC_LFWhlSkid_flg"
  Divide1/1 -> Switch3/3  "VVMC_LFCal4WhlSpdSlideRate_pct"
  [VINP_LFRawWhlSpeed_kph] -> Add5/1
  [VVMC_LFPreVehSpd_kph] -> Add1/2
  Switch2/1 -> Divide1/3
  Relational Operator2/1 -> Switch2/2
  Divide/1 -> FirstOrderFilter/1
  [VVMC_LFWhlCalAcc_Gps] -> Add9/1
  [VVMC_LFPreVehSpd_kph] -> Relational Operator2/1
  Constant5/1 -> Relational Operator2/2
  Add9/1 -> Relational Operator/1
  Switch3/1 -> [VVMC_LF4WhlSpdSlideRate_pct]  "VVMC_LF4WhlSpdSlideRate_pct"
  Relational Operator/1 -> SR_Latch/1
  Add1/1 -> Divide1/1
  Delay7/1 -> Add10/2
  Constant7/1 -> Divide1/2
  [VVMC_LFPreVehSpd_kph] -> Switch2/3
  [VINP_LFRawWhlSpeed_kph] -> Add1/1
  Delay1/1 -> Add5/2
  [VINP_LFRawWhlSpeed_kph] -> Relational Operator3/1
  [task_time_s] -> Divide/3
  Constant25/1 -> Divide/4
  Constant24/1 -> Divide/2
  [VINP_LFRawWhlSpeed_kph] -> Delay1/1
  Add5/1 -> Divide/1
  FirstOrderFilter/1 -> [VVMC_LFWhlCalAcc_Gps]  "VVMC_LFWhlCalAcc_Gps"
  Constant48/1 -> OR1/2
  Constant44/1 -> Product3/2
  Switch10/1 -> [VVMC_LFPreVehSpd_kph]  "VVMC_LFPreVehSpd_kph"
  Constant47/1 -> Equal1/2
  Product2/1 -> Switch10/1
  OR1/1 -> Switch/2
  Equal1/1 -> OR/2
  Constant46/1 -> Equal/2
  Product1/1 -> Add/1  "VVMC_LFDeltaVehSpd_mps"
  Saturation/1 -> Add/2
  [VTQD_GearActualPosn_enum] -> Equal1/1
  Delay/1 -> Product/1
  [VINP_LFRawWhlSpeed_kph] -> Switch10/3
  [VTQD_GearActualPosn_enum] -> Equal/1
  OR/1 -> Switch10/2
  [VVMC_4WheelLongAcc_Gps] -> Product1/1
  Product3/1 -> Switch/1
  Delay5/1 -> Product3/1
  Product/1 -> Switch/3
  Switch/1 -> Saturation/1  "VVMC_LFLastPreVehSpd_mps"
  Constant2/1 -> Product2/2
  Equal/1 -> OR/1
  Constant1/1 -> Product1/2
  Constant11/1 -> Product/2
  [task_time_s] -> Product1/3
  Add/1 -> Product2/1  "VVMC_LFCalPreVehSpd_mps"
  [VVMC_LFPreVehSpd_kph] -> Delay5/1
  [VINP_LFRawWhlSpeed_kph] -> Delay/1
  [VVMC_LFPreVehSpd_kph] -> Delay6/1
  VVMC_4WheelLongAcc_Gps/1 -> [VVMC_4WheelLongAcc_Gps]
  task_time_s/1 -> [task_time_s]
  VINP_LFRawWhlSpeed_kph/1 -> [VINP_LFRawWhlSpeed_kph]
  [VVMC_LFWhlSkid_flg] -> OR1/1
  VTQD_GearActualPosn_enum/1 -> [VTQD_GearActualPosn_enum]
  [VVMC_LFPreVehSpd_kph] -> VVMC_LFPreVehSpd_kph/1
  [VVMC_LFWhlSkid_flg] -> VVMC_LFWhlSkid_flg/1
  [VVMC_LF4WhlSpdSlideRate_pct] -> VVMC_LF4WhlSpdSlideRate_pct/1
  OR2/1 -> SR_Latch/2  "VVMC_LFWhlSkidReset_flg"
  AND1/1 -> OR2/2
  Relational Operator1/1 -> OR2/1
  Constant3/1 -> Relational Operator1/2
  [VINP_LFRawWhlSpeed_kph] -> Relational Operator1/1

== system vmc/VMC/VMC/Slide Rate  Calculation/4Wheel Calculation/LR Wheel ==
  VVMC_4WheelLongAcc_Gps : Inport
  task_time_s : Inport  Port=2
  VINP_LRRawWhlSpeed_kph : Inport  Port=3
  VTQD_GearActualPosn_enum : Inport  Port=4
  AND3 : Logic  Inputs=3  AllPortsSameDT=off  OutDataTypeStr=boolean
  Abs2 : Abs
  Add : Sum
  Add{4,7,13..14} (4 alike) : Sum  Inputs=+-
  Constant1 : Constant  Value=GRAVITY_G
  Constant11 : Constant  Value=KPH2MPS
  Constant19 : Constant  Value=ONE_PERCENT
  Constant2 : Constant  Value=MPS2KPH
  Constant20 : Constant  Value=KVMC_RawWhlSpeedDeadZone_kph
  Constant21 : Constant  Value=ZERO_FLOAT
  Constant22 : Constant  Value=KVMC_RawWhlSpeedDeadZone_kph
  Constant23 : Constant  Value=ONE_FLOAT
  Constant30 : Constant  Value=KPH2MPS
  Constant31 : Constant  Value=GRAVITY_G
  Constant32 : Constant  Value=KVMC_WhlSpdCalAccTs_c
  Constant40 : Constant  Value=KVMC_WheelSkidAccDev_Gps
  Constant41 : Constant  Value=KVMC_SkidRecVehSpdDev_kph
  Constant44 : Constant  Value=KPH2MPS
  Constant46 : Constant  Value=ENUM_GEARACTUALPOSN_D
  Constant47 : Constant  Value=ENUM_GEARACTUALPOSN_R
  Constant48 : Constant  Value=KVMC_PreVehSpdCalSW_flg
  Constant5 : Constant  Value=KVMC_4WheelEnSkidDetSpd_kph
  Constant50 : Constant  Value=KVMC_LRWhlSkidReset_flg
  Delay{,3,5,10..11,16} (6 alike) : Delay  DelayLength=1
  Divide4 : Product  Inputs=*//
  Divide6 : Product  Inputs=**//
  Equal : RelationalOperator  Operator===  OutDataTypeStr=boolean  RndMeth=Simplest
  Equal1 : RelationalOperator  Operator===  OutDataTypeStr=boolean  RndMeth=Simplest
  FirstOrderFilter2 : hcu_lib/Basic_Blocks/FirstOrderFilter
  OR : Logic  Operator=OR  AllPortsSameDT=off  OutDataTypeStr=boolean
  OR1 : Logic  Operator=OR  AllPortsSameDT=off  OutDataTypeStr=boolean
  OR2 : Logic  Operator=OR  AllPortsSameDT=off  OutDataTypeStr=boolean
  Product : Product
  Product1 : Product  Inputs=3
  Product2 : Product
  Product3 : Product
  Relational Operator12 : RelationalOperator  Operator=>  OutDataTypeStr=boolean  RndMeth=Simplest
  Relational Operator{2,7..8,13} (4 alike) : RelationalOperator  Operator=<=  OutDataTypeStr=boolean  RndMeth=Simplest
  SR_Latch2 : hcu_lib/Basic_Blocks/SR_Latch
  Saturation : Saturate  UpperLimit=KVMC_PredVehSpdLimit_mps  LowerLimit=ZERO_FLOAT
  Switch{,7..8,10} (4 alike) : Switch  Criteria=u2 > Threshold
  VVMC_LRPreVehSpd_kph : Outport
  VVMC_LRWhlSkid_flg : Outport  Port=2
  VVMC_LR4WhlSpdSlideRate_pct : Outport  Port=3
  wires:
  Delay3/1 -> Add7/2
  Delay10/1 -> Add13/1
  Constant30/1 -> Divide6/2
  [task_time_s] -> Divide6/3
  Constant41/1 -> Relational Operator13/2
  Constant50/1 -> AND3/3
  Constant31/1 -> Divide6/4
  [VINP_LRRawWhlSpeed_kph] -> Delay11/1
  SR_Latch2/1 -> [VVMC_LRWhlSkid_flg]  "VVMC_LRWhlSkid_flg"
  [VVMC_LRWhlSkid_flg] -> Delay16/1
  Relational Operator13/1 -> AND3/1
  Abs2/1 -> Relational Operator13/1
  Delay16/1 -> AND3/2
  Add7/1 -> Divide6/1
  Relational Operator12/1 -> SR_Latch2/1
  Delay11/1 -> Add13/2
  [VINP_LRRawWhlSpeed_kph] -> Add7/1
  [VINP_LRRawWhlSpeed_kph] -> Delay3/1
  [VVMC_LRWhlCalAcc_Gps] -> Add14/1
  Constant32/1 -> FirstOrderFilter2/3
  FirstOrderFilter2/1 -> [VVMC_LRWhlCalAcc_Gps]  "VVMC_LRWhlCalAcc_Gps"
  Divide6/1 -> FirstOrderFilter2/1
  [VVMC_4WheelLongAcc_Gps] -> Add14/2
  Constant40/1 -> Relational Operator12/2
  Add13/1 -> Abs2/1
  Add14/1 -> Relational Operator12/1
  [task_time_s] -> FirstOrderFilter2/2
  [VVMC_LRPreVehSpd_kph] -> Delay5/1
  [task_time_s] -> Product1/3
  [VVMC_4WheelLongAcc_Gps] -> Product1/1
  Constant44/1 -> Product3/2
  Switch/1 -> Saturation/1  "VVMC_LRLastPreVehSpd_mps"
  Product2/1 -> Switch10/1
  Constant11/1 -> Product/2
  Add/1 -> Product2/1  "VVMC_LRCalPreVehSpd_mps"
  Equal/1 -> OR/1
  [VTQD_GearActualPosn_enum] -> Equal/1
  [VINP_LRRawWhlSpeed_kph] -> Switch10/3
  Constant1/1 -> Product1/2
  Product3/1 -> Switch/1
  Switch10/1 -> [VVMC_LRPreVehSpd_kph]  "VVMC_LRPreVehSpd_kph"
  [VINP_LRRawWhlSpeed_kph] -> Delay/1
  OR1/1 -> Switch/2
  Constant48/1 -> OR1/2
  Constant47/1 -> Equal1/2
  Equal1/1 -> OR/2
  [VTQD_GearActualPosn_enum] -> Equal1/1
  Constant46/1 -> Equal/2
  Constant2/1 -> Product2/2
  Product1/1 -> Add/1  "VVMC_LRDeltaVehSpd_mps"
  Delay/1 -> Product/1
  Product/1 -> Switch/3
  Delay5/1 -> Product3/1
  Saturation/1 -> Add/2
  OR/1 -> Switch10/2
  [VVMC_LRWhlSkid_flg] -> OR1/1
  [VVMC_LRPreVehSpd_kph] -> Delay10/1
  Constant22/1 -> Relational Operator7/2
  [VINP_LRRawWhlSpeed_kph] -> Add4/1
  [VINP_LRRawWhlSpeed_kph] -> Relational Operator8/1
  Relational Operator7/1 -> Switch7/2
  [VVMC_LRPreVehSpd_kph] -> Relational Operator7/1
  Constant19/1 -> Divide4/2
  Switch8/1 -> [VVMC_LR4WhlSpdSlideRate_pct]  "VVMC_LR4WhlSpdSlideRate_pct"
  Constant23/1 -> Switch7/1
  [VVMC_LRPreVehSpd_kph] -> Add4/2
  Constant20/1 -> Relational Operator8/2
  Constant21/1 -> Switch8/1
  Divide4/1 -> Switch8/3  "VVMC_LRCal4WhlSpdSlideRate_pct"
  Switch7/1 -> Divide4/3
  [VVMC_LRPreVehSpd_kph] -> Switch7/3
  Add4/1 -> Divide4/1
  Relational Operator8/1 -> Switch8/2
  task_time_s/1 -> [task_time_s]
  VVMC_4WheelLongAcc_Gps/1 -> [VVMC_4WheelLongAcc_Gps]
  VINP_LRRawWhlSpeed_kph/1 -> [VINP_LRRawWhlSpeed_kph]
  VTQD_GearActualPosn_enum/1 -> [VTQD_GearActualPosn_enum]
  [VVMC_LRPreVehSpd_kph] -> VVMC_LRPreVehSpd_kph/1
  [VVMC_LRWhlSkid_flg] -> VVMC_LRWhlSkid_flg/1
  [VVMC_LR4WhlSpdSlideRate_pct] -> VVMC_LR4WhlSpdSlideRate_pct/1
  [VINP_LRRawWhlSpeed_kph] -> Relational Operator2/1
  Relational Operator2/1 -> OR2/1
  Constant5/1 -> Relational Operator2/2
  AND3/1 -> OR2/2
  OR2/1 -> SR_Latch2/2  "VVMC_LRWhlSkidReset_flg"

== system vmc/VMC/VMC/Slide Rate  Calculation/4Wheel Calculation/RF Wheel ==
  VVMC_4WheelLongAcc_Gps : Inport
  task_time_s : Inport  Port=2
  VINP_RFRawWhlSpeed_kph : Inport  Port=3
  VTQD_GearActualPosn_enum : Inport  Port=4
  AND2 : Logic  Inputs=3  AllPortsSameDT=off  OutDataTypeStr=boolean
  Abs1 : Abs
  Add : Sum
  Add{2,6,11..12} (4 alike) : Sum  Inputs=+-
  Constant1 : Constant  Value=GRAVITY_G
  Constant10 : Constant  Value=ONE_PERCENT
  Constant11 : Constant  Value=KPH2MPS
  Constant12 : Constant  Value=KVMC_RawWhlSpeedDeadZone_kph
  Constant13 : Constant  Value=ZERO_FLOAT
  Constant2 : Constant  Value=MPS2KPH
  Constant27 : Constant  Value=KPH2MPS
  Constant28 : Constant  Value=GRAVITY_G
  Constant29 : Constant  Value=KVMC_WhlSpdCalAccTs_c
  Constant3 : Constant  Value=KVMC_RawWhlSpeedDeadZone_kph
  Constant38 : Constant  Value=KVMC_WheelSkidAccDev_Gps
  Constant39 : Constant  Value=KVMC_SkidRecVehSpdDev_kph
  Constant4 : Constant  Value=ONE_FLOAT
  Constant44 : Constant  Value=KPH2MPS
  Constant46 : Constant  Value=ENUM_GEARACTUALPOSN_D
  Constant47 : Constant  Value=ENUM_GEARACTUALPOSN_R
  Constant48 : Constant  Value=KVMC_PreVehSpdCalSW_flg
  Constant5 : Constant  Value=KVMC_4WheelEnSkidDetSpd_kph
  Constant51 : Constant  Value=KVMC_RFWhlSkidReset_flg
  Delay{,2,5,8..9,15} (6 alike) : Delay  DelayLength=1
  Divide2 : Product  Inputs=*//
  Divide5 : Product  Inputs=**//
  Equal : RelationalOperator  Operator===  OutDataTypeStr=boolean  RndMeth=Simplest
  Equal1 : RelationalOperator  Operator===  OutDataTypeStr=boolean  RndMeth=Simplest
  FirstOrderFilter1 : hcu_lib/Basic_Blocks/FirstOrderFilter
  OR : Logic  Operator=OR  AllPortsSameDT=off  OutDataTypeStr=boolean
  OR1 : Logic  Operator=OR  AllPortsSameDT=off  OutDataTypeStr=boolean
  OR2 : Logic  Operator=OR  AllPortsSameDT=off  OutDataTypeStr=boolean
  Product : Product
  Product1 : Product  Inputs=3
  Product2 : Product
  Product3 : Product
  Relational Operator{1..2,4,11} (4 alike) : RelationalOperator  Operator=<=  OutDataTypeStr=boolean  RndMeth=Simplest
  Relational Operator10 : RelationalOperator  Operator=>  OutDataTypeStr=boolean  RndMeth=Simplest
  SR_Latch1 : hcu_lib/Basic_Blocks/SR_Latch
  Saturation : Saturate  UpperLimit=KVMC_PredVehSpdLimit_mps  LowerLimit=ZERO_FLOAT
  Switch{,1,4,10} (4 alike) : Switch  Criteria=u2 > Threshold
  VVMC_RFPreVehSpd_kph : Outport
  VVMC_RFWhlSkid_flg : Outport  Port=2
  VVMC_RF4WhlSpdSlideRate_pct : Outport  Port=3
  wires:
  [VVMC_4WheelLongAcc_Gps] -> Add12/2
  Switch1/1 -> Divide2/3
  Relational Operator11/1 -> AND2/1
  Divide5/1 -> FirstOrderFilter1/1
  Constant12/1 -> Relational Operator4/2
  Add12/1 -> Relational Operator10/1
  [VINP_RFRawWhlSpeed_kph] -> Add6/1
  Constant13/1 -> Switch4/1
  [VINP_RFRawWhlSpeed_kph] -> Delay2/1
  Constant3/1 -> Relational Operator1/2
  Delay15/1 -> AND2/2
  [VVMC_RFWhlSkid_flg] -> Delay15/1
  Constant27/1 -> Divide5/2
  Relational Operator1/1 -> Switch1/2
  Constant28/1 -> Divide5/4
  Add11/1 -> Abs1/1
  Constant38/1 -> Relational Operator10/2
  Divide2/1 -> Switch4/3  "VVMC_RFCal4WhlSpdSlideRate_pct"
  Delay8/1 -> Add11/1
  [VINP_RFRawWhlSpeed_kph] -> Delay9/1
  Abs1/1 -> Relational Operator11/1
  [task_time_s] -> FirstOrderFilter1/2
  Delay9/1 -> Add11/2
  Constant39/1 -> Relational Operator11/2
  Constant4/1 -> Switch1/1
  Relational Operator4/1 -> Switch4/2
  Constant51/1 -> AND2/3
  Add6/1 -> Divide5/1
  Constant10/1 -> Divide2/2
  [VINP_RFRawWhlSpeed_kph] -> Add2/1
  [VINP_RFRawWhlSpeed_kph] -> Relational Operator4/1
  Relational Operator10/1 -> SR_Latch1/1
  SR_Latch1/1 -> [VVMC_RFWhlSkid_flg]  "VVMC_RFWhlSkid_flg"
  [VVMC_RFWhlCalAcc_Gps] -> Add12/1
  Constant29/1 -> FirstOrderFilter1/3
  FirstOrderFilter1/1 -> [VVMC_RFWhlCalAcc_Gps]  "VVMC_RFWhlCalAcc_Gps"
  Switch4/1 -> [VVMC_RF4WhlSpdSlideRate_pct]  "VVMC_RF4WhlSpdSlideRate_pct"
  Add2/1 -> Divide2/1
  Delay2/1 -> Add6/2
  [task_time_s] -> Divide5/3
  Product/1 -> Switch/3
  Delay5/1 -> Product3/1
  Product3/1 -> Switch/1
  [VVMC_RFPreVehSpd_kph] -> Delay5/1
  [VINP_RFRawWhlSpeed_kph] -> Delay/1
  OR/1 -> Switch10/2
  [VTQD_GearActualPosn_enum] -> Equal/1
  [VINP_RFRawWhlSpeed_kph] -> Switch10/3
  [VTQD_GearActualPosn_enum] -> Equal1/1
  Delay/1 -> Product/1
  Saturation/1 -> Add/2
  Constant2/1 -> Product2/2
  Product1/1 -> Add/1  "VVMC_RFDeltaVehSpd_mps"
  Equal1/1 -> OR/2
  Constant46/1 -> Equal/2
  OR1/1 -> Switch/2
  Constant47/1 -> Equal1/2
  Constant48/1 -> OR1/2
  Switch10/1 -> [VVMC_RFPreVehSpd_kph]  "VVMC_RFPreVehSpd_kph"
  Constant1/1 -> Product1/2
  Product2/1 -> Switch10/1
  Constant11/1 -> Product/2
  Switch/1 -> Saturation/1  "VVMC_RFLastPreVehSpd_mps"
  Constant44/1 -> Product3/2
  [VVMC_4WheelLongAcc_Gps] -> Product1/1
  [task_time_s] -> Product1/3
  Equal/1 -> OR/1
  Add/1 -> Product2/1  "VVMC_RFCalPreVehSpd_mps"
  [VVMC_RFWhlSkid_flg] -> OR1/1
  [VVMC_RFPreVehSpd_kph] -> Delay8/1
  [VVMC_RFPreVehSpd_kph] -> Add2/2
  [VVMC_RFPreVehSpd_kph] -> Relational Operator1/1
  [VVMC_RFPreVehSpd_kph] -> Switch1/3
  VTQD_GearActualPosn_enum/1 -> [VTQD_GearActualPosn_enum]
  VINP_RFRawWhlSpeed_kph/1 -> [VINP_RFRawWhlSpeed_kph]
  VVMC_4WheelLongAcc_Gps/1 -> [VVMC_4WheelLongAcc_Gps]
  task_time_s/1 -> [task_time_s]
  [VVMC_RFPreVehSpd_kph] -> VVMC_RFPreVehSpd_kph/1
  [VVMC_RFWhlSkid_flg] -> VVMC_RFWhlSkid_flg/1
  [VVMC_RF4WhlSpdSlideRate_pct] -> VVMC_RF4WhlSpdSlideRate_pct/1
  Constant5/1 -> Relational Operator2/2
  Relational Operator2/1 -> OR2/1
  [VINP_RFRawWhlSpeed_kph] -> Relational Operator2/1
  AND2/1 -> OR2/2
  OR2/1 -> SR_Latch1/2  "VVMC_RFWhlSkidReset_flg"
